simulink model "Simul20230325"  (R2022a)
settings: Solver=VariableStepAuto  StartTime=0.0  StopTime=40  RelTol=1e-3
settings Model: Creator=aghersin  LastModifiedBy=aghersin

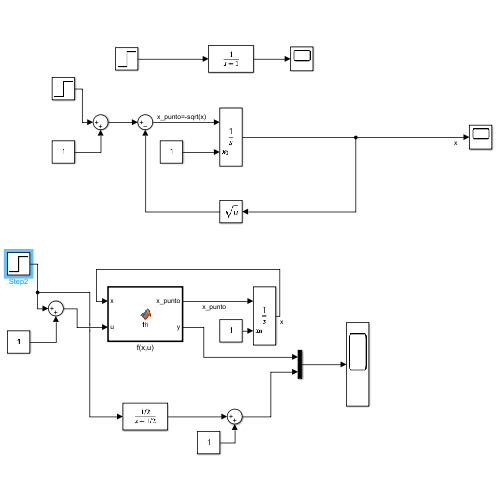
[thumbnail: Simulink's stored preview of the top-level diagram]
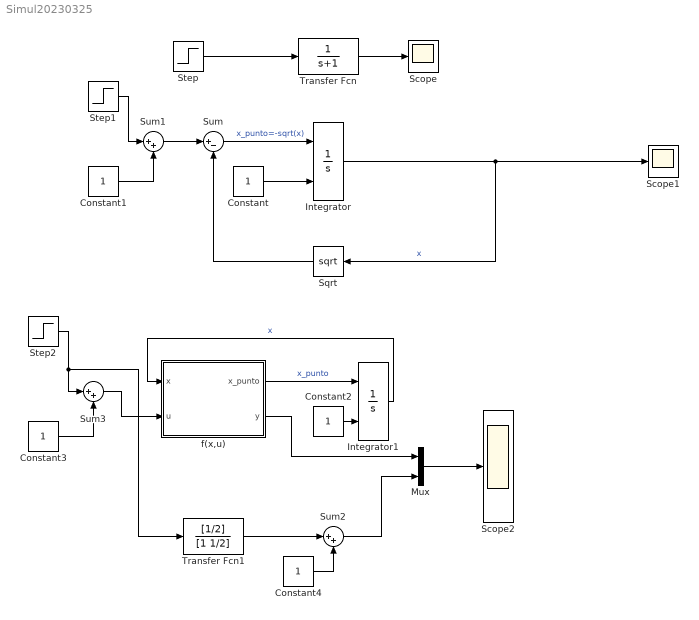
== system Simul20230325 ==
  Constant{,1..4} (5 alike) : Constant
  Integrator : Integrator  InitialConditionSource=external
  Integrator1 : Integrator  InitialConditionSource=external
  Mux : Mux  Inputs=2
  Scope : Scope
  Scope1 : Scope
  Scope2 : Scope
  Sqrt : Sqrt
  Step : Step  SampleTime=0
  Step1 : Step  After=.2  SampleTime=0
  Step2 : Step  After=.1  SampleTime=0
  Sum : Sum  Inputs=|+-
  Sum1 : Sum  Inputs=|++
  Sum2 : Sum  Inputs=|++
  Sum3 : Sum  Inputs=|++
  Transfer Fcn : TransferFcn  Denominator=[1 1]
  Transfer Fcn1 : TransferFcn  Numerator=[1/2]  Denominator=[1 1/2]
  f(x,u) : MATLAB Function  TreatAsAtomicUnit=on
  wires:
  Transfer Fcn/1 -> Scope/1
  Step/1 -> Transfer Fcn/1
  Integrator/1 -> Sqrt/1, Scope1/1  "x"
  Sqrt/1 -> Sum/2
  Constant/1 -> Integrator/2
  Sum/1 -> Integrator/1  "x_punto=-sqrt(x)"
  Sum1/1 -> Sum/1
  Constant1/1 -> Sum1/2
  Step1/1 -> Sum1/1
  Step2/1 -> Sum3/1, Transfer Fcn1/1
  Constant3/1 -> Sum3/2
  Sum3/1 -> f(x,u)/2(u)
  Constant2/1 -> Integrator1/2
  Integrator1/1 -> f(x,u)/1(x)  "x"
  f(x,u)/1(x_punto) -> Integrator1/1  "x_punto"
  Mux/1 -> Scope2/1
  Transfer Fcn1/1 -> Sum2/1
  Sum2/1 -> Mux/2
  Constant4/1 -> Sum2/2
  f(x,u)/2(y) -> Mux/1

== matlab function Simul20230325/f(x,u) ==
  data: x input; u input; x_punto output; y output
function [x_punto,y] = fh(x,u)
x_punto=-sqrt(x)+u;
y=sqrt(x);
